simulink model "Problem5"  (R2020b)
settings: Solver=VariableStepAuto  StartTime=0.0  StopTime=10.0  RelTol=1e-3
model workspace (MAT data in the model file):
  C = Simulink.Parameter
  C.Value = 0.01
  C.DataType = 'auto'
  C.Dimensions = [1 1]
  R = Simulink.Parameter
  R.Value = 10
  R.DataType = 'auto'
  R.Dimensions = [1 1]
settings Model: Creator=ASUS  LastModifiedBy=ASUS

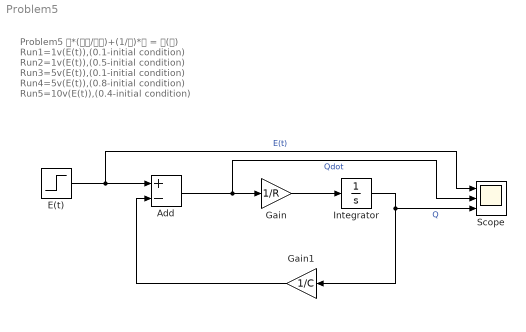
== system Problem5 ==
  note: Problem5
      | 𝑅*(𝑑𝑄/𝑑𝑡)+(1/𝐶)*𝑄 = 𝐸(𝑡)
      |
      | Run1=1v(E(t)),(0.1-initial condition)
      | Run2=1v(E(t)),(0.5-initial condition)
      | Run3=5v(E(t)),(0.1-initial condition)
      | Run4=5v(E(t)),(0.8-initial condition)
      | Run5=10v(E(t)),(0.4-initial condition)
  Add : Sum  Inputs=+-
  E(t) : Step  SampleTime=0
  Gain : Gain  Gain=1/R
  Gain1 : Gain  Gain=1/C
  Integrator : Integrator  InitialCondition=0.5
  Scope : Scope  NumInputPorts=3
  wires:
  E(t)/1 -> Scope/1, Add/1  "E(t)"
  Add/1 -> Scope/2, Gain/1  "Qdot"
  Gain/1 -> Integrator/1
  Integrator/1 -> Scope/3, Gain1/1  "Q"
  Gain1/1 -> Add/2
